simulink model "model"  (R2021a)
settings: Solver=VariableStepAuto  StartTime=0.0  StopTime=5  RelTol=1e-3
InitFcn:
  | clc, clear all, close all
  | addpath('package');
  | 
  | params;
  | load('package/AeroDB.mat');
values from neighbouring files (symbols this model uses):
  Iyy = 44.3618    [linearization.m]    (also in trim.m)
  Mass = 56.2951    [linearization.m]    (also in trim.m)
  Refa = 0.01824    [linearization.m]    (also in trim.m)
  Refl = 0.1524    [linearization.m]    (also in trim.m)
  V = MachTrim * SoS    [linearization.m]    (also in trim.m = cMach * SoS)
undefined symbols (not defined in the file or in its folder): h, tblCM0, tblCMd, tblCMq, tblCz0, tblCzd
libraries: aerolibatmos2 x1
settings Model: Creator=Joshua  LastModifiedBy=Joshua

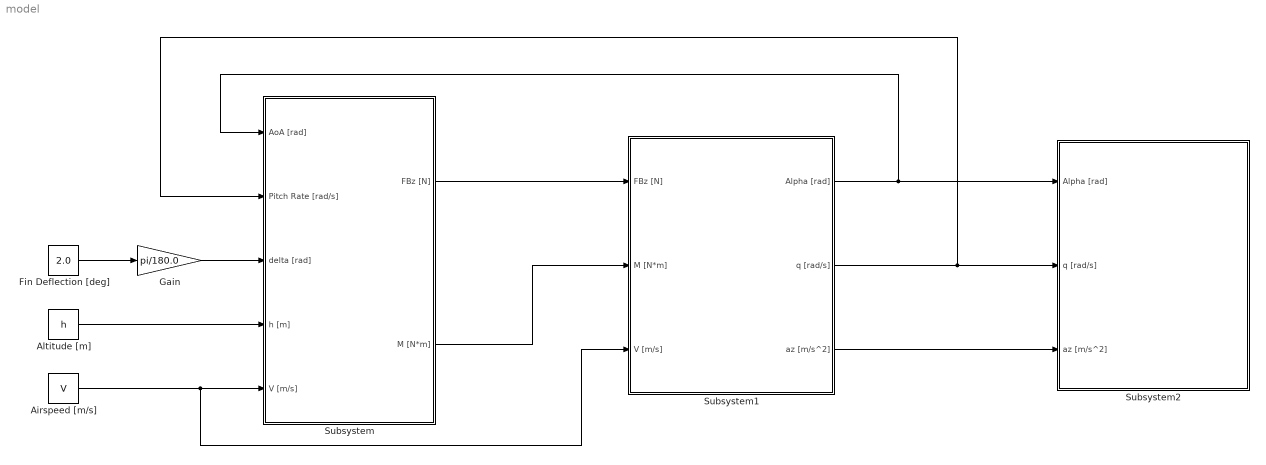
== system model ==
  Airspeed [m/s] : Constant  Value=V
  Altitude [m] : Constant  Value=h
  Fin Deflection [deg] : Constant  Value=2.0
  Gain : Gain  Gain=pi/180.0
  Subsystem : Subsystem
  Subsystem1 : Subsystem
  Subsystem2 : Subsystem
  wires:
  Fin Deflection [deg]/1 -> Gain/1
  Airspeed [m/s]/1 -> Subsystem1/3(V [m/s]), Subsystem/5(V [m/s])
  Gain/1 -> Subsystem/3(delta [rad])
  Altitude [m]/1 -> Subsystem/4(h [m])
  Subsystem/1(FBz [N]) -> Subsystem1/1(FBz [N])
  Subsystem/2(M [N*m]) -> Subsystem1/2(M [N*m])
  Subsystem1/1(Alpha [rad]) -> Subsystem/1(AoA [rad]), Subsystem2/1(Alpha [rad])
  Subsystem1/2(q [rad/s]) -> Subsystem/2(Pitch Rate [rad/s]), Subsystem2/2(q [rad/s])
  Subsystem1/3(az [m/s^2]) -> Subsystem2/3(az [m/s^2])

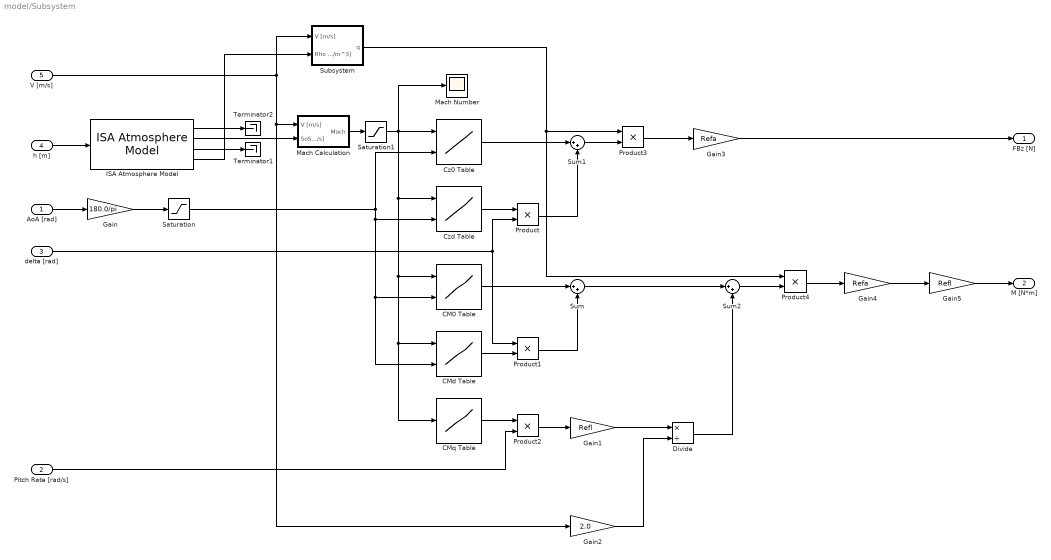
== system model/Subsystem ==
  AoA [rad] : Inport
  Pitch Rate [rad/s] : Inport  Port=2
  delta [rad] : Inport  Port=3
  h [m] : Inport  Port=4
  V [m/s] : Inport  Port=5
  CM0 Table : Lookup_n-D  LookupTableObject=tblCz0  BreakpointsForDimension1=[1:14]  BreakpointsForDimension2=[1:15]  Table=tblCM0  InternalRulePriority=Speed  RndMeth=Simplest  InputSameDT=on
      settings: InputPortMap=u0,u1
  CMd Table : Lookup_n-D  LookupTableObject=tblCz0  BreakpointsForDimension1=[1:14]  BreakpointsForDimension2=[1:15]  Table=tblCMd  InternalRulePriority=Speed  RndMeth=Simplest  InputSameDT=on
      settings: InputPortMap=u0,u1
  CMq Table : Lookup_n-D  NumberOfTableDimensions=1  LookupTableObject=tblCz0  BreakpointsForDimension1=[1:14]  BreakpointsForDimension2=[1:15]  Table=tblCMq  InternalRulePriority=Speed  RndMeth=Simplest  InputSameDT=on
  Cz0 Table : Lookup_n-D  LookupTableObject=tblCz0  BreakpointsForDimension1=[1:14]  BreakpointsForDimension2=[1:15]  Table=tblCz0  InternalRulePriority=Speed  RndMeth=Simplest  InputSameDT=on
      settings: InputPortMap=u0,u1
  Czd Table : Lookup_n-D  LookupTableObject=tblCz0  BreakpointsForDimension1=[1:14]  BreakpointsForDimension2=[1:15]  Table=tblCzd  InternalRulePriority=Speed  RndMeth=Simplest  InputSameDT=on
      settings: InputPortMap=u0,u1
  Divide : Product  Inputs=*/
  Gain : Gain  Gain=180.0/pi
  Gain1 : Gain  Gain=Refl
  Gain2 : Gain  Gain=2.0
  Gain3 : Gain  Gain=Refa
  Gain4 : Gain  Gain=Refa
  Gain5 : Gain  Gain=Refl
  ISA Atmosphere Model : aerolibatmos2/ISA Atmosphere Model  custom=off  g=9.80665  gamma=1.4  R=287.0531  L=0.0065  h_trop=11000  h_strat=20000  rho0=1.225  P0=101325  T0=288.15  h0=0
  Mach Calculation : Subsystem
  Mach Number : Scope
  Product{,1..4} (5 alike) : Product
  Saturation : Saturate  UpperLimit=180  LowerLimit=-180
  Saturation1 : Saturate  UpperLimit=25  LowerLimit=0
  Subsystem : Subsystem
  Sum : Sum  Inputs=|++
  Sum1 : Sum  Inputs=|++
  Sum2 : Sum  Inputs=|++
  Terminator1 : Terminator
  Terminator2 : Terminator
  FBz [N] : Outport
  M [N*m] : Outport  Port=2
  wires:
  Gain/1 -> Saturation/1
  AoA [rad]/1 -> Gain/1
  h [m]/1 -> ISA Atmosphere Model/1
  ISA Atmosphere Model/3 -> Terminator1/1
  V [m/s]/1 -> Subsystem/1(V [m/s]), Mach Calculation/1(V [m/s]), Gain2/1
  ISA Atmosphere Model/4 -> Subsystem/2(Rho [kg/m^3])
  ISA Atmosphere Model/2 -> Mach Calculation/2(SoS [m/s])
  ISA Atmosphere Model/1 -> Terminator2/1
  Mach Calculation/1(Mach) -> Saturation1/1
  Saturation/1 -> CMd Table/2, CM0 Table/2, Czd Table/2, Cz0 Table/2
  Czd Table/1 -> Product/1
  delta [rad]/1 -> Product/2, Product1/1
  CMd Table/1 -> Product1/2
  CMq Table/1 -> Product2/1
  Pitch Rate [rad/s]/1 -> Product2/2
  Product1/1 -> Sum/2
  CM0 Table/1 -> Sum/1
  Product/1 -> Sum1/2
  Cz0 Table/1 -> Sum1/1
  Sum1/1 -> Product3/2
  Subsystem/1(q) -> Product4/1, Product3/1
  Product2/1 -> Gain1/1
  Gain1/1 -> Divide/1
  Gain2/1 -> Divide/2
  Sum/1 -> Sum2/1
  Divide/1 -> Sum2/2
  Sum2/1 -> Product4/2
  Product3/1 -> Gain3/1
  Product4/1 -> Gain4/1
  Gain4/1 -> Gain5/1
  Gain5/1 -> M [N*m]/1
  Gain3/1 -> FBz [N]/1
  Saturation1/1 -> Mach Number/1, CM0 Table/1, CMd Table/1, CMq Table/1, Czd Table/1, Cz0 Table/1

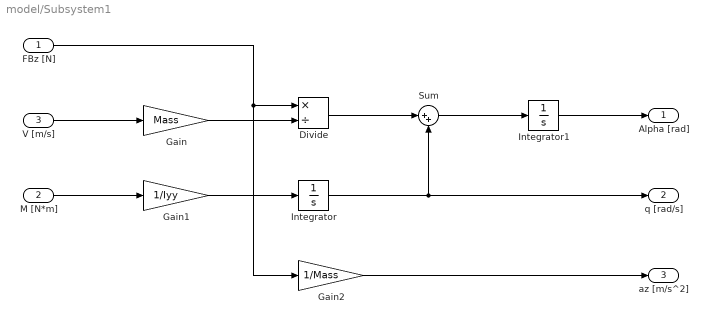
== system model/Subsystem1 ==
  FBz [N] : Inport
  M [N*m] : Inport  Port=2
  V [m/s] : Inport  Port=3
  Divide : Product  Inputs=*/
  Gain : Gain  Gain=Mass
  Gain1 : Gain  Gain=1/Iyy
  Gain2 : Gain  Gain=1/Mass
  Integrator : Integrator
  Integrator1 : Integrator
  Sum : Sum  Inputs=|++
  Alpha [rad] : Outport
  q [rad/s] : Outport  Port=2
  az [m/s^2] : Outport  Port=3
  wires:
  Gain/1 -> Divide/2
  V [m/s]/1 -> Gain/1
  M [N*m]/1 -> Gain1/1
  FBz [N]/1 -> Gain2/1, Divide/1
  Gain1/1 -> Integrator/1
  Integrator/1 -> q [rad/s]/1, Sum/2
  Sum/1 -> Integrator1/1
  Divide/1 -> Sum/1
  Integrator1/1 -> Alpha [rad]/1
  Gain2/1 -> az [m/s^2]/1

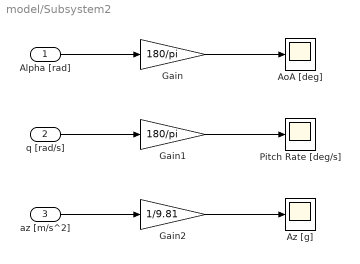
== system model/Subsystem2 ==
  Alpha [rad] : Inport
  q [rad/s] : Inport  Port=2
  az [m/s^2] : Inport  Port=3
  AoA [deg] : Scope
  Az [g] : Scope
  Gain : Gain  Gain=180/pi
  Gain1 : Gain  Gain=180/pi
  Gain2 : Gain  Gain=1/9.81
  Pitch Rate [deg/s] : Scope
  wires:
  az [m/s^2]/1 -> Gain2/1
  q [rad/s]/1 -> Gain1/1
  Alpha [rad]/1 -> Gain/1
  Gain/1 -> AoA [deg]/1
  Gain1/1 -> Pitch Rate [deg/s]/1
  Gain2/1 -> Az [g]/1

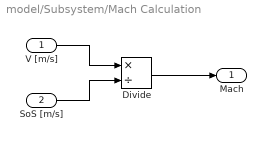
== system model/Subsystem/Mach Calculation ==
  V [m/s] : Inport
  SoS [m/s] : Inport  Port=2
  Divide : Product  Inputs=*/
  Mach : Outport
  wires:
  V [m/s]/1 -> Divide/1
  SoS [m/s]/1 -> Divide/2
  Divide/1 -> Mach/1

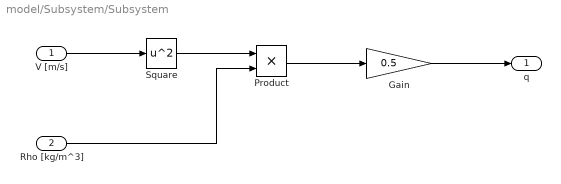
== system model/Subsystem/Subsystem ==
  V [m/s] : Inport
  Rho [kg/m^3] : Inport  Port=2
  Gain : Gain  Gain=0.5
  Product : Product
  Square : Math  Operator=square  SaturateOnIntegerOverflow=on
  q : Outport
  wires:
  V [m/s]/1 -> Square/1
  Square/1 -> Product/1
  Rho [kg/m^3]/1 -> Product/2
  Product/1 -> Gain/1
  Gain/1 -> q/1
